simulink model "problem2"  (R2020b)
settings: Solver=VariableStepAuto  StartTime=0.0  StopTime=10.0  RelTol=1e-3
undefined symbols (not defined in the file): b
settings Model: Creator=Pulkit Khandelwal  LastModifiedBy=Pulkit Khandelwal

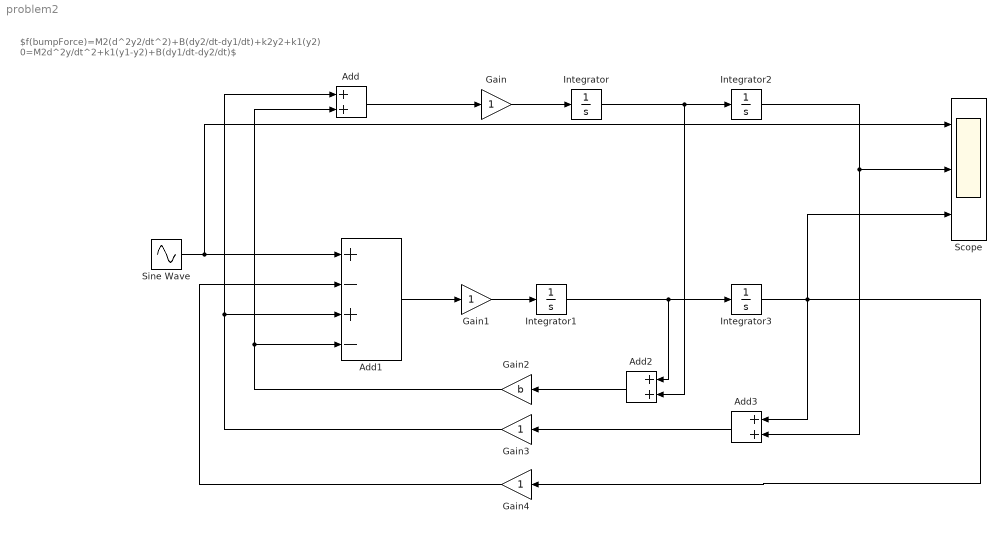
== system problem2 ==
  note: $f(bumpForce)=M2(d^2y2/dt^2)+B(dy2/dt-dy1/dt)+k2y2+k1(y2) 0=M2d^2y/dt^2+k1(y1-y2)+B(dy1/dt-dy2/dt)$
  Add : Sum
  Add1 : Sum  Inputs=+-+-
  Add2 : Sum
  Add3 : Sum
  Gain{,1,3..4} (4 alike) : Gain
  Gain2 : Gain  Gain=b
  Integrator{,1..3} (4 alike) : Integrator
  Scope : Scope  NumInputPorts=3
  Sine Wave : Sin  SampleTime=0
  wires:
  Add/1 -> Gain/1
  Gain/1 -> Integrator/1
  Integrator/1 -> Add2/2, Integrator2/1
  Add1/1 -> Gain1/1
  Gain1/1 -> Integrator1/1
  Integrator1/1 -> Add2/1, Integrator3/1
  Add2/1 -> Gain2/1
  Add3/1 -> Gain3/1
  Gain2/1 -> Add1/4, Add/2
  Gain3/1 -> Add1/3, Add/1
  Gain4/1 -> Add1/2
  Integrator3/1 -> Scope/3, Add3/1, Gain4/1
  Integrator2/1 -> Add3/2, Scope/2
  Sine Wave/1 -> Scope/1, Add1/1
